simulink model "psdRange_model"  (R2020b)
settings: Solver=ode1  StartTime=0.0  StopTime=10.0  RelTol=1e-3
settings Model: Creator=leonk  LastModifiedBy=leonk

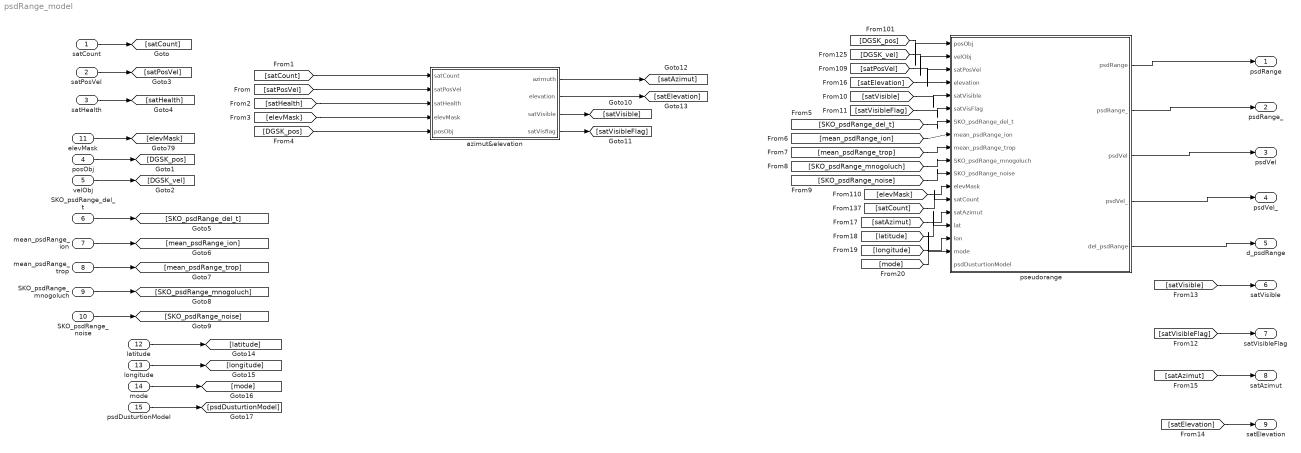
== system psdRange_model ==
  satCount : Inport
  satPosVel : Inport  Port=2  PortDimensions=[6,32]  Interpolate=off
  satHealth : Inport  Port=3  PortDimensions=32  Interpolate=off
  posObj : Inport  Port=4
  velObj : Inport  Port=5
  SKO_psdRange_del_t : Inport  Port=6
  mean_psdRange_ion : Inport  Port=7
  mean_psdRange_trop : Inport  Port=8
  SKO_psdRange_mnogoluch : Inport  Port=9
  SKO_psdRange_noise : Inport  Port=10
  elevMask : Inport  Port=11
  latitude : Inport  Port=12
  longitude : Inport  Port=13
  mode : Inport  Port=14
  psdDusturtionModel : Inport  Port=15
  azimut&elevation : MATLAB Function  TreatAsAtomicUnit=on
  pseudorange : MATLAB Function  TreatAsAtomicUnit=on
  psdRange : Outport  PortDimensions=32
  psdRange_ : Outport  Port=2  PortDimensions=32
  psdVel : Outport  Port=3  PortDimensions=32
  psdVel_ : Outport  Port=4  PortDimensions=32
  d_psdRange : Outport  Port=5  PortDimensions=32
  satVisible : Outport  Port=6
  satVisibleFlag : Outport  Port=7
  satAzimut : Outport  Port=8
  satElevation : Outport  Port=9
  wires:
  [elevMask] -> azimut&elevation/4(elevMask)
  satPosVel/1 -> [satPosVel]
  mean_psdRange_trop/1 -> [mean_psdRange_trop]
  [mean_psdRange_trop] -> pseudorange/9(mean_psdRange_trop)
  mean_psdRange_ion/1 -> [mean_psdRange_ion]
  [SKO_psdRange_mnogoluch] -> pseudorange/10(SKO_psdRange_mnogoluch)
  SKO_psdRange_del_t/1 -> [SKO_psdRange_del_t]
  [SKO_psdRange_noise] -> pseudorange/11(SKO_psdRange_noise)
  SKO_psdRange_noise/1 -> [SKO_psdRange_noise]
  [satCount] -> pseudorange/13(satCount)
  azimut&elevation/1(azimuth) -> [satAzimut]
  [DGSK_vel] -> pseudorange/2(velObj)
  velObj/1 -> [DGSK_vel]
  [DGSK_pos] -> pseudorange/1(posObj)
  [satHealth] -> azimut&elevation/3(satHealth)
  [satPosVel] -> pseudorange/3(satPosVel)
  azimut&elevation/4(satVisflag) -> [satVisibleFlag]
  elevMask/1 -> [elevMask]
  [satPosVel] -> azimut&elevation/2(satPosVel)
  pseudorange/2(psdRange_) -> psdRange_/1
  pseudorange/1(psdRange) -> psdRange/1
  satHealth/1 -> [satHealth]
  [SKO_psdRange_del_t] -> pseudorange/7(SKO_psdRange_del_t)
  satCount/1 -> [satCount]
  SKO_psdRange_mnogoluch/1 -> [SKO_psdRange_mnogoluch]
  [elevMask] -> pseudorange/12(elevMask)
  azimut&elevation/3(satVisible) -> [satVisible]
  posObj/1 -> [DGSK_pos]
  [satCount] -> azimut&elevation/1(satCount)
  [mean_psdRange_ion] -> pseudorange/8(mean_psdRange_ion)
  [DGSK_pos] -> azimut&elevation/5(posObj)
  [satVisible] -> pseudorange/5(satVisible)
  [satVisibleFlag] -> pseudorange/6(satVisFlag)
  [satVisible] -> satVisible/1
  [satVisibleFlag] -> satVisibleFlag/1
  pseudorange/4(psdVel_) -> psdVel_/1
  pseudorange/5(del_psdRange) -> d_psdRange/1
  pseudorange/3(psdVel) -> psdVel/1
  [satAzimut] -> satAzimut/1
  [satElevation] -> satElevation/1
  azimut&elevation/2(elevation) -> [satElevation]
  [satElevation] -> pseudorange/4(elevation)
  [satAzimut] -> pseudorange/14(satAzimut)
  [latitude] -> pseudorange/15(lat)
  [longitude] -> pseudorange/16(lon)
  [mode] -> pseudorange/17(mode)
  mode/1 -> [mode]
  longitude/1 -> [longitude]
  latitude/1 -> [latitude]
  psdDusturtionModel/1 -> [psdDusturtionModel]

== matlab function psdRange_model/pseudorange ==
  data: posObj input size=3; psdRange output size=32; velObj input size=3; satPosVel input size=6,32; elevation input size=32; satVisible input; satVisFlag input uint8 size=32; psdRange_ output size=32; psdVel output size=32; psdVel_ output size=32; SKO_psdRange_del_t input; mean_psdRange_ion input; mean_psdRange_trop input; SKO_psdRange_mnogoluch input; SKO_psdRange_noise input; elevMask input; satCount input; del_psdRange output; satAzimut input; lat input; lon input; mode input; psdDusturtionModel input
function [psdRange, psdRange_, psdVel, psdVel_, del_psdRange] = pseudorange(...
    posObj, velObj, satPosVel, elevation, satVisible, satVisFlag,   ...
    SKO_psdRange_del_t, mean_psdRange_ion, mean_psdRange_trop, SKO_psdRange_mnogoluch,...
    SKO_psdRange_noise, elevMask, satCount, satAzimut, lat, lon, mode, psdDusturtionModel)
    
    psdRange     = zeros(32, 1);
    psdRange_    = zeros(32, 1);
    psdVel       = zeros(32, 1);
    psdVel_      = zeros(32, 1);
    del_psdRange = zeros(32, 1);
    
    for ii = 1:satCount
        if satVisFlag(ii) > 0.5
            %дальность до НКА:
            psdRange(ii) = sqrt(  (posObj(1) - satPosVel(1,ii)).^2 ... 
                                + (posObj(2) - satPosVel(2,ii)).^2 ...
                                + (posObj(3) - satPosVel(3,ii)).^2 );
                        
            %псевдодальность (расчет и добавление погрешности):
            
%             
%             psdR_del_T    = (randn()/5)*SKO_psdRange_del_t;
%             psdRMnogoluch = (randn()/5)*SKO_psdRange_mnogoluch;
%             psdRNoise     = (randn()/5)*SKO_psdRange_noise;
%             psdRTrop      = abs((mean_psdRange_trop * 0.707) / sin(elevation(ii)));
%             psdRIon       = abs((mean_psdRange_ion  * 0.707) / sin(elevation(ii)));
%             del_psdRange(ii)  = psdR_del_T + psdRMnogoluch + psdRTrop + psdRIon + psdRNoise; %%%%
%             psdRange_(ii)     = psdRange(ii) + del_psdRange(ii);

            %Use DO-229 PSD error model
            sigm_URA  = 5.7;% [м]
            Re = 6378136; h = 350000;
            sigm_UIRE = sqrt((1 - ( Re*cos(elevation(ii)) / (Re + h))));
            %submath for URIE psd err
                psi = (0.0137 / (elevation(ii) + 0.11)) + 0.022;
                phi = lat + psi * cos( satAzimut(ii) );
                if     phi >  0.416 
                    phi = 0.416;
                elseif phi < -0.416 
                    phi = -0.416; 
                end
                lambda = lon + (psi * sin( satAzimut(ii) ) / cos( phi ));
                phi_m = rad2deg((phi + 0.064*cos(lambda - 1.617)) * (3.14 / 2));
                if     phi_m >= 55 
                    tau_2 = 36;
                elseif phi_m <= 20 
                    tau_2 = 81;
                else
                    tau_2 = 20.25;
                end
            sigm_UIRE = sigm_UIRE * sqrt(tau_2);
            sigm_AIR  = sqrt( (0.13 + 0.53*exp(-elevation(ii) / deg2rad(10))) + 0.36^2);           
            sigm_TRP = ( 0.12 * ( 1.001 / sqrt( 0.002001 + sin( elevation(ii) )^2 ) ) );
            
            del_psdRange(ii)  = sqrt(sigm_URA^2 + sigm_UIRE^2 + sigm_AIR^2  + sigm_TRP^2) * mode;
            if psdDusturtionModel % if 0 - DO229STYLE (left&right gaussian model, 1 - REALSTYLE only right gaussian side)
                del_psdRange = abs(del_psdRange);
            end
            psdRange_(ii)     = psdRange(ii) + (randn(1) / 4) * del_psdRange(ii);  %fuuuck matlab randn(1)/5 = 1 SKO                         %%%%
            
                
            %псевдоскорость
            psdVel(ii) =   (((satPosVel(1,ii) - posObj(1)) .* (satPosVel(4,ii) - velObj(1))) + ...
                           ( (satPosVel(2,ii) - posObj(2)) .* (satPosVel(5,ii) - velObj(2))) + ...
                           ( (satPosVel(3,ii) - posObj(3)) .* (satPosVel(6,ii) - velObj(3))))./ psdRange(ii);
            psdVel_(ii)  = (((satPosVel(1,ii) - posObj(1)) .* (satPosVel(4,ii) - velObj(1))) + ...
                           ( (satPosVel(2,ii) - posObj(2)) .* (satPosVel(5,ii) - velObj(2))) + ...
                           ( (satPosVel(3,ii) - posObj(3)) .* (satPosVel(6,ii) - velObj(3))))./ psdRange_(ii);
            
        end
    end
end

== matlab function psdRange_model/azimut&elevation ==
  data: azimuth output size=32 [0..32]; satCount input; elevation output size=32; satVisible output uint8; satPosVel input size=[6,32]; satHealth input size=32; elevMask input; posObj input size=3; satVisflag output uint8 size=32
function [azimuth, elevation,satVisible,satVisflag] = pseudorange(satCount, satPosVel, satHealth,elevMask, posObj)
  
    elevMask = deg2rad(elevMask);
    
    elevation  = zeros(32,1);
    azimuth    = zeros(32,1);
    satVisflag = uint8(zeros(32,1));
    satVisible = uint8(zeros(1,1));
    
    posX = posObj(1);
    posY = posObj(2);
    posZ = posObj(3);
    
    R_g = sqrt(posX^2 + posY^2);
    R   = sqrt(posX^2 + posY^2 + posZ^2);
    
    A_see_flag      = zeros(3,3);
    A_see_flag(1,1) = - posY / R_g;
    A_see_flag(1,2) =   posX / R_g;
    A_see_flag(2,1) = -(posX * posZ) / (R_g * R);
    A_see_flag(2,2) = -(posY * posZ) / (R_g * R);
    A_see_flag(2,3) =   R_g / R;
    A_see_flag(3,1) =   posX / R_g;
    A_see_flag(3,2) =   posY / R_g;
    A_see_flag(3,3) =   posZ / R_g;
      
    for ii = 1:satCount
        
        R_s__r = zeros(3,1);
        
        R_s__r(1,1) = satPosVel(1,ii) - posX;
        R_s__r(2,1) = satPosVel(2,ii) - posY;
        R_s__r(3,1) = satPosVel(3,ii) - posZ;
        R_s_r = A_see_flag * R_s__r;
    
        if R_g == 0
            error('Углы неопределены');
        end
        
        sin_El = R_s_r(3) / sqrt(R_s_r(1)^2 + R_s_r(2)^2 + R_s_r(3)^2);
        cos_El = sqrt(1 - sin_El^2);
        
        if sin_El == 1
            elevation(ii) = pi/2;
        else
            elevation(ii) = atan(sin_El / cos_El);
        end
        if R_s_r(2) == 0
            if R_s_r(1) > 0
                azimuth(ii) = pi/2;
            else
                azimuth(ii) = 3*pi/2;
            end
        else
            azimuth(ii) = atan (R_s_r(1) / R_s_r(2));
        end
        if R_s_r(2) < 0
            azimuth(ii) = azimuth(ii) + pi;
        else
            azimuth(ii) = azimuth(ii) + 2 * pi;
        end     
        if  elevation(ii) < elevMask || satHealth(ii) > 0.5
            azimuth(ii) = NaN;
            elevation(ii) = NaN;
            satVisflag(ii) = int8(0);
        else
            satVisflag(ii) = int8(1);
        end
    end
    satVisible = uint8(sum(satVisflag));
end
% 
% function pos = getDGSK(lat, lon, alt)
% 
%     pos = zeros(3,1);
% 
%     b = 6356751.3618;
%     a = 63784136;
%     e2    = double(0.0066943662); 
% 
%     N = (a^2) ./ sqrt(1-e2*(sin(lat).^2));
% 
%     X = (N + alt)*cos(lat)*cos(lon);
%     Y = (N + alt)*cos(lat)*sin(lon);
%     Z = (((b^2)/(a^2))*N + alt)*sin(alt);
%     
%     pos = [X,Y,Z];
%     
% end
